simulink model "simulaTrajetoria"  (R2023b)
settings: Solver=VariableStepAuto  StartTime=0.0  StopTime=60  RelTol=1e-4
values from neighbouring files (symbols this model uses):
  alpha_k = constantes(14)    [calculaMatrizesModelo.m]    (also in simulaModeloSimulink.m; simulaTrajetoriaSimulink.m)
  alpha_s = constantes(13)    [calculaMatrizesModelo.m]    (also in simulaModeloSimulink.m; simulaTrajetoriaSimulink.m)
  b = constantes(7)    [calculaMatrizesModelo.m]    (also in simulaModeloSimulink.m; simulaTrajetoriaSimulink.m)
  d = constantes(5)    [calculaMatrizesModelo.m]    (also in simulaModeloSimulink.m; simulaTrajetoriaSimulink.m)
  f_k = constantes(12)    [calculaMatrizesModelo.m]    (also in simulaModeloSimulink.m; simulaTrajetoriaSimulink.m)
  f_s = constantes(11)    [calculaMatrizesModelo.m]    (also in simulaModeloSimulink.m; simulaTrajetoriaSimulink.m)
  g = 9.81    [calculaMatrizesModelo.m]    (also in simulaModeloSimulink.m; simulaTrajetoriaSimulink.m)
  i_sp = i_sp+1    [ddmr.m]    (also in simulaTrajetoriaSimulink.m = 1)
  K_ce = constantes(8)    [calculaMatrizesModelo.m]    (also in simulaModeloSimulink.m; simulaTrajetoriaSimulink.m)
  k_i = constantes(15)    [calculaMatrizesModelo.m]    (also in simulaModeloSimulink.m; simulaTrajetoriaSimulink.m)
  k_p = constantes(16)    [calculaMatrizesModelo.m]    (also in simulaModeloSimulink.m; simulaTrajetoriaSimulink.m)
  K_t = constantes(9)    [calculaMatrizesModelo.m]    (also in simulaModeloSimulink.m; simulaTrajetoriaSimulink.m)
  L = constantes(2)    [calculaMatrizesModelo.m]    (also in simulaModeloSimulink.m; simulaTrajetoriaSimulink.m)
  m = m_c + 2*m_w    [calculaMatrizesModelo.m]    (also in simulaModeloSimulink.m; simulaTrajetoriaSimulink.m)
  m_c = constantes(3)    [calculaMatrizesModelo.m]    (also in simulaModeloSimulink.m; simulaTrajetoriaSimulink.m)
  Md = (4*I_w^2*L^2 + 2*m*I_w*L^2*R^2 + 2*I_t*I_w*R^2 + I_t*m*R^4)    [simulaModeloSimulink.m]    (also in simulaTrajetoriaSimulink.m)
  Mn1 = (m*L^2*R^2 + 4*I_w*L^2 + I_t*R^2)/(4*I_w^2*L^2 + 2*m*I_w*L^2*R^2 + 2*I_t*I_w*R^2 + I_t*m*R^4)    [simulaModeloSimulink.m]    (also in simulaTrajetoriaSimulink.m)
  Mn2 = (R^2*(- m*L^2 + I_t))    [simulaModeloSimulink.m]    (also in simulaTrajetoriaSimulink.m)
  N = constantes(6)    [calculaMatrizesModelo.m]    (also in simulaModeloSimulink.m; simulaTrajetoriaSimulink.m)
  N_sp = size(setpoints,1)    [ddmr.m]    (also in simulaTrajetoriaSimulink.m)
  R = 0.034    [calculaErros.m]    (also in calculaMatrizesModelo.m = constantes(1); plotTrajetoria.m = 0.175; simulaModeloSimulink.m = constantes(1); simulaTrajetoriaSimulink.m = constantes(1))
  R_a = constantes(10)    [calculaMatrizesModelo.m]    (also in simulaModeloSimulink.m; simulaTrajetoriaSimulink.m)
  setpoints = reshape(setpoints,[],1)    [simulaTrajetoriaSimulink.m]    (also in testes2.m = readmatrix('../SETPOINTS/'+trajetoria+'.csv'))
  T = 1e-2    (= 0.01)    [otimizaControladorOnline.m]    (also in otimizaModelo.m = tempos(2)-tempos(1); otimizaModeloOffline.m; simulaModeloSimulink.m = tempo(2)-tempo(1); simulaTrajetoria.m)
undefined symbols (not defined in the file or in its folder): magnitude
libraries: slpidlib x2, simulink x2, fuzblock x1
settings Model: Creator=Gabriel Sousa  LastModifiedBy=Gabriel Sousa

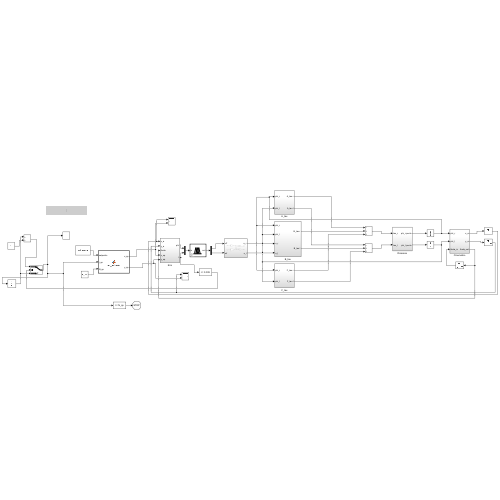
[thumbnail: Simulink's stored preview of the top-level diagram]
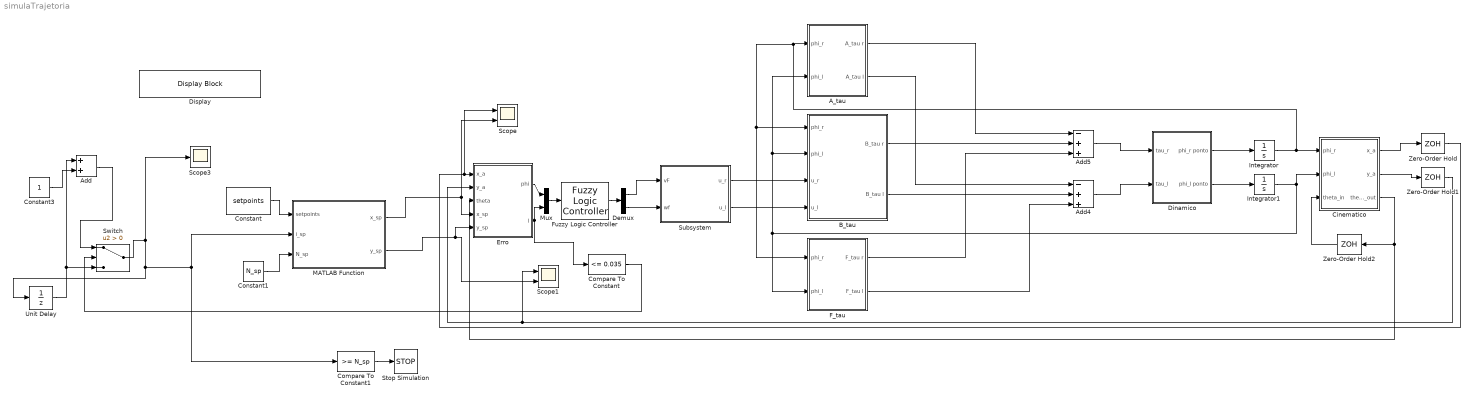
== system simulaTrajetoria ==
  A_tau : Subsystem
  Add : Sum
  Add4 : Sum  Inputs=-++
  Add5 : Sum  Inputs=-++
  B_tau : Subsystem
  Cinematico : Subsystem
  Compare To Constant : simulink/Logic and Bit Operations/Compare To Constant  relop=<=  const=0.035  OutDataTypeStr=boolean
  Compare To Constant1 : simulink/Logic and Bit Operations/Compare To Constant  relop=>=  const=N_sp  OutDataTypeStr=boolean
  Constant : Constant  Value=setpoints  VectorParams1D=off
  Constant1 : Constant  Value=N_sp
  Constant3 : Constant
  Demux : Demux  Outputs=2
  Dinamico : Subsystem
  Display : DisplayBlock  LabelPosition=Hide  Transparency=1
  Erro : Subsystem
  F_tau : Subsystem
  Fuzzy Logic Controller : fuzblock/Fuzzy Logic  Controller  FIS=fis  OutputSampleNumber=101  DataType=double  FuzzifiedInputs=off  RuleFiringStrengths=off  RuleOutputs=off  AggregatedOutputs=off  SimulateUsing=Interpreted execution  OutOfRangeInputValueMessage=warning  NoRuleFiredMessage=warning  EmptyOutputFuzzySetMessage=warning
  Integrator : Integrator
  Integrator1 : Integrator
  MATLAB Function : MATLAB Function  TreatAsAtomicUnit=on
  Mux : Mux  Inputs=2
  Scope : Scope  NumInputPorts=2
  Scope1 : Scope  NumInputPorts=2
  Scope3 : Scope
  Stop Simulation : Stop
  Subsystem : Subsystem
  Switch : Switch  Criteria=u2 > Threshold  SaturateOnIntegerOverflow=off  InputSameDT=off
  Unit Delay : UnitDelay  InitialCondition=i_sp  SampleTime=T  HasFrameUpgradeWarning=on
  Zero-Order Hold : ZeroOrderHold  SampleTime=T
  Zero-Order Hold1 : ZeroOrderHold  SampleTime=T
  Zero-Order Hold2 : ZeroOrderHold  SampleTime=T
  wires:
  Fuzzy Logic Controller/1 -> Demux/1
  Demux/1 -> Subsystem/1(vF)
  Demux/2 -> Subsystem/2(wf)
  Mux/1 -> Fuzzy Logic Controller/1
  Erro/1(phi) -> Mux/1
  Erro/2(l) -> Mux/2, Compare To Constant/1
  MATLAB Function/1(x_sp) -> Erro/4(x_sp), Scope/2
  MATLAB Function/2(y_sp) -> Scope1/2, Erro/5(y_sp)
  Constant/1 -> MATLAB Function/1(setpoints)
  Compare To Constant/1 -> Switch/2
  Constant3/1 -> Add/2
  Add/1 -> Switch/1
  Unit Delay/1 -> Add/1, Switch/3
  Switch/1 -> Unit Delay/1, MATLAB Function/2(i_sp), Compare To Constant1/1, Scope3/1
  Constant1/1 -> MATLAB Function/3(N_sp)
  Compare To Constant1/1 -> Stop Simulation/1
  Cinematico/3(theta_out) -> Zero-Order Hold2/1, Erro/3(theta)
  Add5/1 -> Dinamico/1(tau_r)
  Dinamico/2(phi_l ponto) -> Integrator1/1
  Subsystem/2(u_l) -> B_tau/4(u_l)
  Zero-Order Hold2/1 -> Cinematico/3(theta_in)
  A_tau/2(A_tau l) -> Add4/1
  Integrator1/1 -> B_tau/2(phi_l), A_tau/2(phi_l), F_tau/2(phi_l), Cinematico/2(phi_l)
  Integrator/1 -> Cinematico/1(phi_r), F_tau/1(phi_r), B_tau/1(phi_r), A_tau/1(phi_r)
  Subsystem/1(u_r) -> B_tau/3(u_r)
  Cinematico/2(y_a) -> Zero-Order Hold1/1
  B_tau/2(B_tau l) -> Add4/2
  Dinamico/1(phi_r ponto) -> Integrator/1
  A_tau/1(A_tau r) -> Add5/1
  F_tau/2(F_tau l) -> Add4/3
  F_tau/1(F_tau r) -> Add5/3
  Add4/1 -> Dinamico/2(tau_l)
  B_tau/1(B_tau r) -> Add5/2
  Cinematico/1(x_a) -> Zero-Order Hold/1
  Zero-Order Hold/1 -> Scope/1, Erro/1(x_a)
  Zero-Order Hold1/1 -> Scope1/1, Erro/2(y_a)

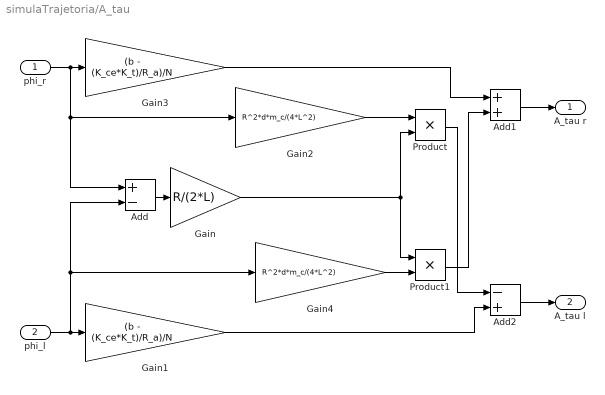
== system simulaTrajetoria/A_tau ==
  phi_r : Inport
  phi_l : Inport  Port=2
  Add : Sum  Inputs=+-
  Add1 : Sum
  Add2 : Sum  Inputs=-+
  Gain : Gain  Gain=R/(2*L)
  Gain1 : Gain  Gain=(b - (K_ce*K_t)/R_a)/N
  Gain2 : Gain  Gain=R^2*d*m_c/(4*L^2)
  Gain3 : Gain  Gain=(b - (K_ce*K_t)/R_a)/N
  Gain4 : Gain  Gain=R^2*d*m_c/(4*L^2)
  Product : Product
  Product1 : Product
  A_tau r : Outport
  A_tau l : Outport  Port=2
  wires:
  phi_r/1 -> Gain2/1, Add/1, Gain3/1
  Gain3/1 -> Add1/1
  Gain1/1 -> Add2/2
  phi_l/1 -> Gain1/1, Gain4/1, Add/2
  Add/1 -> Gain/1
  Gain4/1 -> Product1/2
  Gain/1 -> Product/2, Product1/1
  Gain2/1 -> Product/1
  Product1/1 -> Add1/2
  Product/1 -> Add2/1
  Add2/1 -> A_tau l/1
  Add1/1 -> A_tau r/1

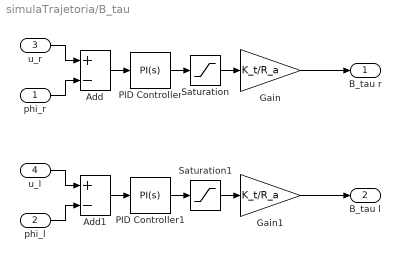
== system simulaTrajetoria/B_tau ==
  phi_r : Inport
  phi_l : Inport  Port=2
  u_r : Inport  Port=3
  u_l : Inport  Port=4
  Add : Sum  Inputs=+-
  Add1 : Sum  Inputs=+-
  Gain : Gain  Gain=K_t/R_a
  Gain1 : Gain  Gain=K_t/R_a
  PID Controller : slpidlib/PID Controller  Controller=PI  Form=Ideal  TimeDomain=Continuous-time  UseExternalTs=off  SampleTime=-1  IntegratorMethod=Forward Euler  FilterMethod=Forward Euler  ControllerParametersSource=internal  P=k_p  I=k_i  UseKiTs=off  D=0  N=100  UseFilter=on  TunerSelectOption=Transfer Function Based (PID Tuner App)  InitialConditionSource=internal  InitialConditionForIntegrator=0  InitialConditionForFilter=0  DifferentiatorICPrevScaledInput=0  ExternalReset=none  TrackingMode=off  Kt=1  LimitOutput=off  SatLimitsSource=internal  UpperSaturationLimit=inf  LowerSaturationLimit=-inf  LinearizeAsGain=on  AntiWindupMode=none  Kb=1  LimitIntegrator=off  UpperIntegratorSaturationLimit=inf  LowerIntegratorSaturationLimit=-inf  POutMin=[]  POutMax=[]  IOutMin=[]  IOutMax=[]  DOutMin=[]  DOutMax=[]  NOutMin=[]  NOutMax=[]  SumOutMin=[]  SumOutMax=[]  SaturationOutMin=[]  SaturationOutMax=[]  PParamMin=[]  PParamMax=[]  IParamMin=[]  IParamMax=[]  DParamMin=[]  DParamMax=[]  NParamMin=[]  NParamMax=[]  KbParamMin=[]  KbParamMax=[]  KtParamMin=[]  KtParamMax=[]  KbOutMin=[]  KbOutMax=[]  KtOutMin=[]  KtOutMax=[]  IntegratorOutMin=[]  IntegratorOutMax=[]  FilterOutMin=[]  FilterOutMax=[]  SumI1OutMin=[]  SumI1OutMax=[]  SumI2OutMin=[]  SumI2OutMax=[]  SumI3OutMin=[]  SumI3OutMax=[]  SumI4OutMin=[]  SumI4OutMax=[]  SumDOutMin=[]  SumDOutMax=[]  DifferentiatorOutMin=[]  DifferentiatorOutMax=[]  FilterDiffOutCoefMin=[]  FilterDiffOutCoefMax=[]  ReciprocalOutMin=[]  ReciprocalOutMax=[]  SumDenOutMin=[]  SumDenOutMax=[]  SumNumOutMin=[]  SumNumOutMax=[]  DivideOutMin=[]  DivideOutMax=[]  UdiffTsProdOutMin=[]  UdiffTsProdOutMax=[]  NTsProdOutMin=[]  NTsProdOutMax=[]  UintegralTsProdOutMin=[]  UintegralTsProdOutMax=[]  UngainTsProdOutMin=[]  UngainTsProdOutMax=[]  ClampingZeroOutDataTypeStr=Inherit: Inherit via back propagation  ClampingZeroOutMin=[]  ClampingZeroOutMax=[]  FilterDenConstantOutDataTypeStr=Inherit: Inherit via back propagation  FilterDenConstantOutMin=[]  FilterDenConstantOutMax=[]  PCopyOutDataTypeStr=Inherit: Inherit via back propagation  PCopyOutMin=[]  PCopyOutMax=[]  NCopyOutDataTypeStr=Inherit: Inherit via back propagation  NCopyOutMin=[]  NCopyOutMax=[]  IntegratorContinuousStateAttributes=''  IntegratorStateMustResolveToSignalObject=off  IntegratorRTWStateStorageClass=Auto  FilterContinuousStateAttributes=''  FilterStateMustResolveToSignalObject=off  FilterRTWStateStorageClass=Auto  ParallelPVariant=Passthrough  IdealPVariant=InternalParameters  IVariant=InternalParameters  DVariant=Disabled  IntegratorVariant=Continuous  SatVariant=Disabled  AWVariant=Passthrough  PCopyVariant=Disabled  TRVariant=Disabled  FdbkBlocksVariant=Forward  IdealPFdbkVariant=Disabled  SatFdbkVariant=Disabled  DerivativeFilterVariant=Disabled  NVariant=Disabled  NCopyVariant=Disabled_SignalSpec  FilterICVariant=Disabled  IntegratorICVariant=InternalICs  ExternalResetVariant=Disabled  TRSumVariant=Passthrough  SumFdbkVariant=Disabled  SumVariant=Sum_PI  TsampFilterVariant=InternalTs  TsampNgainVariant=Passthrough  TsampIntegralVariant=Disabled_SignalSpec  ExternalSaturationOutDataTypeStr=Inherit: Same as second input
  PID Controller1 : slpidlib/PID Controller  Controller=PI  Form=Ideal  TimeDomain=Continuous-time  UseExternalTs=off  SampleTime=-1  IntegratorMethod=Forward Euler  FilterMethod=Forward Euler  ControllerParametersSource=internal  P=k_p  I=k_i  UseKiTs=off  D=0  N=100  UseFilter=on  TunerSelectOption=Transfer Function Based (PID Tuner App)  InitialConditionSource=internal  InitialConditionForIntegrator=0  InitialConditionForFilter=0  DifferentiatorICPrevScaledInput=0  ExternalReset=none  TrackingMode=off  Kt=1  LimitOutput=off  SatLimitsSource=internal  UpperSaturationLimit=inf  LowerSaturationLimit=-inf  LinearizeAsGain=on  AntiWindupMode=none  Kb=1  LimitIntegrator=off  UpperIntegratorSaturationLimit=inf  LowerIntegratorSaturationLimit=-inf  POutMin=[]  POutMax=[]  IOutMin=[]  IOutMax=[]  DOutMin=[]  DOutMax=[]  NOutMin=[]  NOutMax=[]  SumOutMin=[]  SumOutMax=[]  SaturationOutMin=[]  SaturationOutMax=[]  PParamMin=[]  PParamMax=[]  IParamMin=[]  IParamMax=[]  DParamMin=[]  DParamMax=[]  NParamMin=[]  NParamMax=[]  KbParamMin=[]  KbParamMax=[]  KtParamMin=[]  KtParamMax=[]  KbOutMin=[]  KbOutMax=[]  KtOutMin=[]  KtOutMax=[]  IntegratorOutMin=[]  IntegratorOutMax=[]  FilterOutMin=[]  FilterOutMax=[]  SumI1OutMin=[]  SumI1OutMax=[]  SumI2OutMin=[]  SumI2OutMax=[]  SumI3OutMin=[]  SumI3OutMax=[]  SumI4OutMin=[]  SumI4OutMax=[]  SumDOutMin=[]  SumDOutMax=[]  DifferentiatorOutMin=[]  DifferentiatorOutMax=[]  FilterDiffOutCoefMin=[]  FilterDiffOutCoefMax=[]  ReciprocalOutMin=[]  ReciprocalOutMax=[]  SumDenOutMin=[]  SumDenOutMax=[]  SumNumOutMin=[]  SumNumOutMax=[]  DivideOutMin=[]  DivideOutMax=[]  UdiffTsProdOutMin=[]  UdiffTsProdOutMax=[]  NTsProdOutMin=[]  NTsProdOutMax=[]  UintegralTsProdOutMin=[]  UintegralTsProdOutMax=[]  UngainTsProdOutMin=[]  UngainTsProdOutMax=[]  ClampingZeroOutDataTypeStr=Inherit: Inherit via back propagation  ClampingZeroOutMin=[]  ClampingZeroOutMax=[]  FilterDenConstantOutDataTypeStr=Inherit: Inherit via back propagation  FilterDenConstantOutMin=[]  FilterDenConstantOutMax=[]  PCopyOutDataTypeStr=Inherit: Inherit via back propagation  PCopyOutMin=[]  PCopyOutMax=[]  NCopyOutDataTypeStr=Inherit: Inherit via back propagation  NCopyOutMin=[]  NCopyOutMax=[]  IntegratorContinuousStateAttributes=''  IntegratorStateMustResolveToSignalObject=off  IntegratorRTWStateStorageClass=Auto  FilterContinuousStateAttributes=''  FilterStateMustResolveToSignalObject=off  FilterRTWStateStorageClass=Auto  ParallelPVariant=Passthrough  IdealPVariant=InternalParameters  IVariant=InternalParameters  DVariant=Disabled  IntegratorVariant=Continuous  SatVariant=Disabled  AWVariant=Passthrough  PCopyVariant=Disabled  TRVariant=Disabled  FdbkBlocksVariant=Forward  IdealPFdbkVariant=Disabled  SatFdbkVariant=Disabled  DerivativeFilterVariant=Disabled  NVariant=Disabled  NCopyVariant=Disabled_SignalSpec  FilterICVariant=Disabled  IntegratorICVariant=InternalICs  ExternalResetVariant=Disabled  TRSumVariant=Passthrough  SumFdbkVariant=Disabled  SumVariant=Sum_PI  TsampFilterVariant=InternalTs  TsampNgainVariant=Passthrough  TsampIntegralVariant=Disabled_SignalSpec  ExternalSaturationOutDataTypeStr=Inherit: Same as second input
  Saturation : Saturate  UpperLimit=12  LowerLimit=-12
  Saturation1 : Saturate  UpperLimit=12  LowerLimit=-12
  B_tau r : Outport
  B_tau l : Outport  Port=2
  wires:
  Gain/1 -> B_tau r/1
  Add/1 -> PID Controller/1
  PID Controller/1 -> Saturation/1
  Saturation/1 -> Gain/1
  phi_r/1 -> Add/2
  Saturation1/1 -> Gain1/1
  Add1/1 -> PID Controller1/1
  phi_l/1 -> Add1/2
  PID Controller1/1 -> Saturation1/1
  Gain1/1 -> B_tau l/1
  u_r/1 -> Add/1
  u_l/1 -> Add1/1

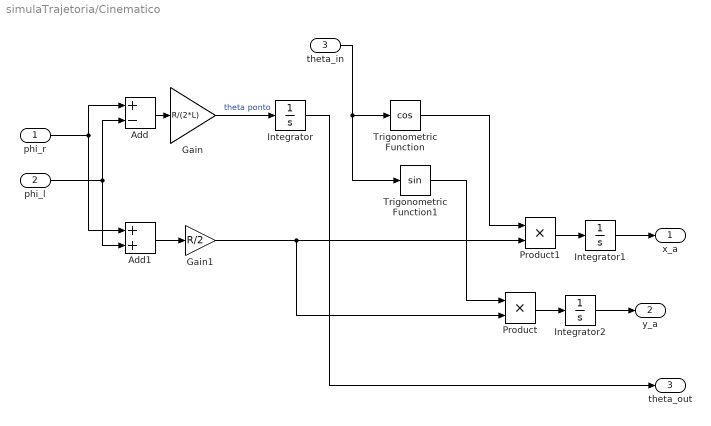
== system simulaTrajetoria/Cinematico ==
  phi_r : Inport
  phi_l : Inport  Port=2
  theta_in : Inport  Port=3
  Add : Sum  Inputs=+-
  Add1 : Sum
  Gain : Gain  Gain=R/(2*L)
  Gain1 : Gain  Gain=R/2
  Integrator : Integrator
  Integrator1 : Integrator
  Integrator2 : Integrator
  Product : Product
  Product1 : Product
  Trigonometric Function : Trigonometry  Operator=cos
  Trigonometric Function1 : Trigonometry
  x_a : Outport  VectorParamsAs1DForOutWhenUnconnected=off
  y_a : Outport  Port=2  VectorParamsAs1DForOutWhenUnconnected=off
  theta_out : Outport  Port=3  VectorParamsAs1DForOutWhenUnconnected=off
  wires:
  phi_r/1 -> Add/1, Add1/1
  phi_l/1 -> Add/2, Add1/2
  Add/1 -> Gain/1
  Gain/1 -> Integrator/1  "theta ponto"
  Add1/1 -> Gain1/1
  Trigonometric Function/1 -> Product1/1
  Trigonometric Function1/1 -> Product/1
  Product/1 -> Integrator2/1
  Product1/1 -> Integrator1/1
  Integrator1/1 -> x_a/1
  Integrator2/1 -> y_a/1
  Gain1/1 -> Product1/2, Product/2
  theta_in/1 -> Trigonometric Function1/1, Trigonometric Function/1
  Integrator/1 -> theta_out/1

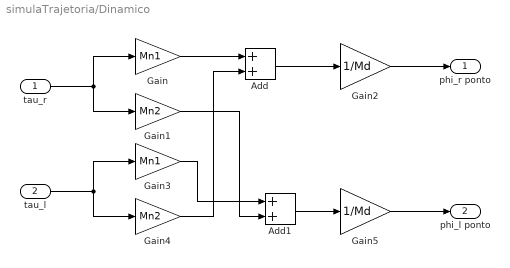
== system simulaTrajetoria/Dinamico ==
  tau_r : Inport
  tau_l : Inport  Port=2
  Add : Sum
  Add1 : Sum
  Gain : Gain  Gain=Mn1
  Gain1 : Gain  Gain=Mn2
  Gain2 : Gain  Gain=1/Md
  Gain3 : Gain  Gain=Mn1
  Gain4 : Gain  Gain=Mn2
  Gain5 : Gain  Gain=1/Md
  phi_r ponto : Outport  VectorParamsAs1DForOutWhenUnconnected=off
  phi_l ponto : Outport  Port=2  VectorParamsAs1DForOutWhenUnconnected=off
  wires:
  tau_r/1 -> Gain/1, Gain1/1
  tau_l/1 -> Gain3/1, Gain4/1
  Gain5/1 -> phi_l ponto/1
  Gain2/1 -> phi_r ponto/1
  Gain/1 -> Add/1
  Gain4/1 -> Add/2
  Gain3/1 -> Add1/1
  Gain1/1 -> Add1/2
  Add1/1 -> Gain5/1
  Add/1 -> Gain2/1

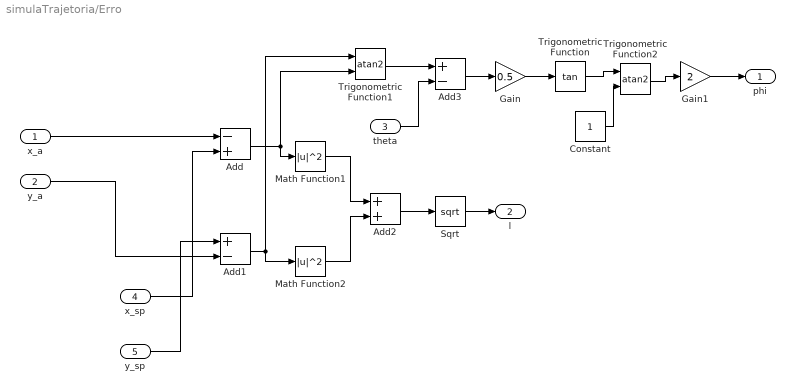
== system simulaTrajetoria/Erro ==
  x_a : Inport
  y_a : Inport  Port=2
  theta : Inport  Port=3
  x_sp : Inport  Port=4
  y_sp : Inport  Port=5
  Add : Sum  Inputs=-+
  Add1 : Sum  Inputs=+-
  Add2 : Sum
  Add3 : Sum  Inputs=+-
  Constant : Constant
  Gain : Gain  Gain=0.5
  Gain1 : Gain  Gain=2
  Math Function1 : Math  Operator=magnitude^2  SignedPower=on
  Math Function2 : Math  Operator=magnitude^2  SignedPower=on
  Sqrt : Sqrt
  Trigonometric Function : Trigonometry  Operator=tan
  Trigonometric Function1 : Trigonometry  Operator=atan2
  Trigonometric Function2 : Trigonometry  Operator=atan2
  phi : Outport  VectorParamsAs1DForOutWhenUnconnected=off
  l : Outport  Port=2
  wires:
  x_a/1 -> Add/1
  x_sp/1 -> Add/2
  y_sp/1 -> Add1/1
  y_a/1 -> Add1/2
  Add1/1 -> Math Function2/1, Trigonometric Function1/1
  Add/1 -> Math Function1/1, Trigonometric Function1/2
  Math Function2/1 -> Add2/2
  Math Function1/1 -> Add2/1
  Add2/1 -> Sqrt/1
  Sqrt/1 -> l/1
  Trigonometric Function1/1 -> Add3/1
  theta/1 -> Add3/2
  Add3/1 -> Gain/1
  Gain1/1 -> phi/1
  Trigonometric Function2/1 -> Gain1/1
  Trigonometric Function/1 -> Trigonometric Function2/1
  Gain/1 -> Trigonometric Function/1
  Constant/1 -> Trigonometric Function2/2

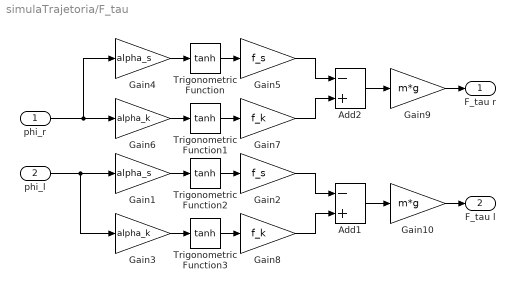
== system simulaTrajetoria/F_tau ==
  phi_r : Inport
  phi_l : Inport  Port=2
  Add1 : Sum  Inputs=-+
  Add2 : Sum  Inputs=-+
  Gain1 : Gain  Gain=alpha_s
  Gain10 : Gain  Gain=m*g
  Gain2 : Gain  Gain=f_s
  Gain3 : Gain  Gain=alpha_k
  Gain4 : Gain  Gain=alpha_s
  Gain5 : Gain  Gain=f_s
  Gain6 : Gain  Gain=alpha_k
  Gain7 : Gain  Gain=f_k
  Gain8 : Gain  Gain=f_k
  Gain9 : Gain  Gain=m*g
  Trigonometric Function{,1..3} (4 alike) : Trigonometry  Operator=tanh
  F_tau r : Outport
  F_tau l : Outport  Port=2
  wires:
  Gain5/1 -> Add2/1
  Trigonometric Function/1 -> Gain5/1
  Gain4/1 -> Trigonometric Function/1
  Gain6/1 -> Trigonometric Function1/1
  Gain7/1 -> Add2/2
  Trigonometric Function1/1 -> Gain7/1
  phi_r/1 -> Gain4/1, Gain6/1
  Trigonometric Function3/1 -> Gain8/1
  Gain1/1 -> Trigonometric Function2/1
  Gain2/1 -> Add1/1
  Gain8/1 -> Add1/2
  Trigonometric Function2/1 -> Gain2/1
  Gain3/1 -> Trigonometric Function3/1
  phi_l/1 -> Gain3/1, Gain1/1
  Add2/1 -> Gain9/1
  Add1/1 -> Gain10/1
  Gain9/1 -> F_tau r/1
  Gain10/1 -> F_tau l/1

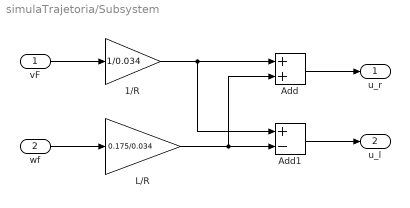
== system simulaTrajetoria/Subsystem ==
  vF : Inport
  wf : Inport  Port=2
  1/R : Gain  Gain=1/0.034
  Add : Sum
  Add1 : Sum  Inputs=+-
  L/R : Gain  Gain=0.175/0.034
  u_r : Outport
  u_l : Outport  Port=2
  wires:
  vF/1 -> 1/R/1
  wf/1 -> L/R/1
  1/R/1 -> Add1/1, Add/1
  L/R/1 -> Add1/2, Add/2
  Add/1 -> u_r/1
  Add1/1 -> u_l/1

== matlab function simulaTrajetoria/MATLAB Function ==
  data: setpoints input; x_sp output; i_sp input; N_sp input; y_sp output
function [x_sp,y_sp] = set_setpoint(setpoints,i_sp,N_sp) %#codegen
% Declaração de tipo de saída


i_sp = int32(i_sp); % Converte i_sp para int32

x_sp = setpoints(i_sp);
y_sp = setpoints(i_sp+N_sp);

end
